simulink model "untitled"  (Simulink 5.0)
settings: Solver=ode3  StartTime=0.0  StopTime=10.0  FixedStep=0.001  RelTol=1e-3
undefined symbols (not defined in the file): Kd, Ki, Kp
settings Model: LastModifiedBy=ENGENHARIA

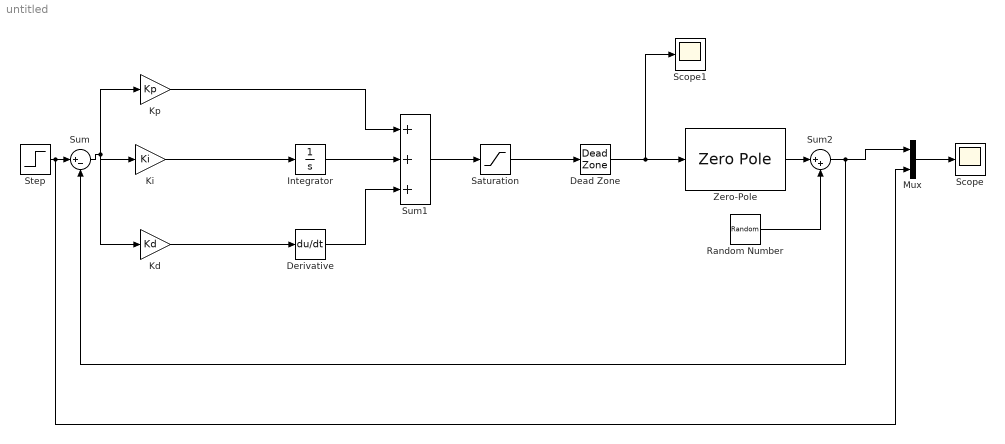
== system untitled ==
  Dead Zone : DeadZone  LowerValue=0  UpperValue=0  SaturateOnIntegerOverflow=on
  Derivative : Derivative
  Integrator : Integrator
  Kd : Gain  Gain=Kd  SaturateOnIntegerOverflow=on
  Ki : Gain  Gain=Ki  SaturateOnIntegerOverflow=on
  Kp : Gain  Gain=Kp  SaturateOnIntegerOverflow=on
  Mux : Mux  Inputs=2
  Random Number : RandomNumber  Variance=0.1  SampleTime=0
  Saturation : Saturate  UpperLimit=5  LowerLimit=0
  Scope : Scope
      settings: SaveName=sinais  DataFormat=Array
  Scope1 : Scope
      settings: TimeRange=10  YMin=-1
  Step : Step  Time=0  After=20  SampleTime=0
  Sum : Sum  Inputs=|+-  SaturateOnIntegerOverflow=on
  Sum1 : Sum  Inputs=+++  SaturateOnIntegerOverflow=on
  Sum2 : Sum  Inputs=|++  SaturateOnIntegerOverflow=on
  Zero-Pole : ZeroPole  Zeros=[]  Poles=[0 -2000 -10]  Gain=[20*2000*10]
  wires:
  Saturation/1 -> Dead Zone/1
  Dead Zone/1 -> Zero-Pole/1, Scope1/1
  Step/1 -> Sum/1, Mux/2
  Kp/1 -> Sum1/1
  Integrator/1 -> Sum1/2
  Ki/1 -> Integrator/1
  Derivative/1 -> Sum1/3
  Kd/1 -> Derivative/1
  Sum/1 -> Kp/1, Kd/1, Ki/1
  Sum1/1 -> Saturation/1
  Mux/1 -> Scope/1
  Zero-Pole/1 -> Sum2/1
  Random Number/1 -> Sum2/2
  Sum2/1 -> Mux/1, Sum/2
